simulink model "DW_MCU_Simulation_Architecture_DualMotor"  (R2018a)
settings: Solver=FixedStepDiscrete  StartTime=0.0  StopTime=20  FixedStep=TimeSteps.ModelStep  RelTol=1e-6
PreLoadFcn:
  | addpath('tools');
  | addpath('tools\Config_UI');
  | addpath('tools\support');
  | addpath('tools\FMIKit_for_Simulink');
  | addpath('tools\FMIKit_for_Simulink\slx');
  | addpath('tools\SpeedCommand');
  | addpath('tools\SpeedCommand\exe');
  | addpath('tools\SpeedCommand\view');
  | addpath('tools\MciAPI');
  | addpath('tools\MciAPI\exe');
  | addpath('tools\MciAPI\exe\enums');
  | addpath('tools\Read_PDB_File');
  | addpath('tools\Read_PDB_File\exe');
  | addpath('tools\PILComm');
  | addpath('tools\PILComm\exe');
  | 
  | addpath('exe');
  | addpath('source\c_code');
  | addpath('source\simulink\PlantModels\Sensor');
  | addpath('source\simulink\PlantModels\Rectifiers');
  | addpath('source\simulink\PlantModels\Motors\CIM');
  | addpath('source\simulink\PlantModels\Motors\BPM');
  | addpath('source\simulink\PlantModels\Motors\BPM\SFunctions\10k\Dyno');
  | addpath('source\simulink\PlantModels\Motors\BPM\SFunctions\10k\HA');
  | addpath('source\simulink\PlantModels\Motors\BPM\SFunctions\10k\VA_Agitation');
  | addpath('source\simulink\PlantModels\Motors\BPM\SFunctions\10k\VA_Spin');
  | addpath('source\simulink\PlantModels\Motors\BPM\SFunctions\16k\Dyno');
  | addpath('source\simulink\PlantModels\Motors\BPM\SFunctions\16k\HA');
  | addpath('source\simulink\PlantModels\Motors\BPM\SFunctions\16k\VA_Agitation');
  | addpath('source\simulink\PlantModels\Motors\BPM\SFunctions\16k\VA_Spin');
  | addpath('source\simulink\PlantModels\Inverter');
  | 
  | 
  | addpath('exported_models');
  | clear all;
  | 
  | try
  | FMIKit.initialize()
  | catch
  | display('FMI Kit Initialization Skipped');
  | end
  | 
  | Sim_Arch_Config_UI_App;
PostLoadFcn:
  | myws = get_param(gcs, 'modelworkspace');
  | myws.clear;
  | clear myws;
  | evalin('base', 'recompile_mcu_sim_arch = 1;');
  | updateModelWS(gcs);
InitFcn:
  | if (evalin('base', 'exist(''smlarch_need_reset'') == 1'))
  |     msgbox('Reload Variables before Running');
  |     set_param(gcs, 'SimulationCommand', 'stop');
  | end
  | BusInit;
  | if(  (exist('SimArchUID')) && (strcmp(SimArchUID, 'a') == 1)  )
  |     updateModelWS(gcs);
  | end
  | useModelWS(gcs);
  | Simulink.sdi.close;
model workspace (MAT data in the model file):
  DC_Bus.Const_Vbus = 325
  InputCircuit.R_line = 0.62
  InputCircuit.L_line = 5e-05
  InputCircuit.C_buscap = 8.2e-05
  InputCircuit.R_diode = 0.22
  InputCircuit.R_buscap = 3.235
  InputCircuit.V_knee = 0.64
  InputCircuit.G_off = 3e-09
  InputCircuit.L_pfc = 0
  InputCircuit.R_pfc = 0
  InputCircuit.Vr = 230
  InputCircuit.Vdc_i = 325
  InputCircuit.freq = 50
  InputCircuit.C1 = -0.6111111111
  InputCircuit.C2 = 1.715258789
  InputCircuit.Cvolt = 0.007695895522
  InputCircuit.Vcc = 3.3
  InputCircuit.ADCBit = 12
  Mechanical.belt_ratio = 10
  Mechanical.JDrum = 0.001
  Mechanical.damp = 0
  Mechanical.m_unb = 0
  Mechanical.r_unb = 0
  Mechanical.M_D = 1
  Mechanical.M = 0.2
  Mechanical.R_Drum = 0.254
  Mechanical.R_J = 0.05
  Mechanical.CF = 0
  Motor.Electrical.Rs_a_Ref = 40.5
  Motor.Electrical.Rs_b_Ref = 40.5
  Motor.Electrical.Rs_c_Ref = 40.5
  Motor.Electrical.p_Pole_Pairs = 1
  Motor.Electrical.PM_Flux_f01 = 0.089
  Motor.Electrical.PM_Flux_f02 = 0
  Motor.Electrical.PM_Flux_f03 = 0
  Motor.Electrical.PM_Flux_f04 = 0
  Motor.Electrical.PM_Flux_f05 = 0
  Motor.Electrical.PM_Flux_f06 = 0
  Motor.Electrical.PM_Flux_f07 = 0
  Motor.Electrical.PM_Flux_f08 = 0
  Motor.Electrical.PM_Flux_f09 = 0
  Motor.Electrical.PM_Flux_f10 = 0
  Motor.Electrical.PM_Flux_f11 = 0
  Motor.Electrical.PM_Flux_f12 = 0
  Motor.Electrical.PM_Flux_f13 = 0
  Motor.Electrical.ajust = 1.57
  Motor.Electrical.alpha_s = 0
  Motor.Mechanical.Jrotor = 2e-05
  Motor.Mechanical.B = 0.0002
  Motor.Mechanical.Jadd = 0
  Motor.Mechanical.Rs_Temperature_Ref = 22
  Motor.Mechanical.PM_Temperature_Ref = 22
  Motor.Mechanical.TR = 1
  Motor.Power_Loss.Rot_Loss_Flag = 0
  Motor.Power_Loss.Rot_Loss_Speed0 = 0
  Motor.Power_Loss.Rot_Loss_Speed1 = 500
  Motor.Power_Loss.Rot_Loss_Speed2 = 3000
  Motor.Power_Loss.Rot_Loss_Speed3 = 4000
  Motor.Power_Loss.Rot_Loss_Speed4 = 4000
  Motor.Power_Loss.Rot_Loss_Speed5 = 4000
  Motor.Power_Loss.Rot_Loss_Speed6 = 4000
  Motor.Power_Loss.Rot_Loss_Speed7 = 4000
  Motor.Power_Loss.Rot_Loss_Power0 = 0
  Motor.Power_Loss.Rot_Loss_Power1 = 0
  Motor.Power_Loss.Rot_Loss_Power2 = 0
  Motor.Power_Loss.Rot_Loss_Power3 = 0
  Motor.Power_Loss.Rot_Loss_Power4 = 0
  Motor.Power_Loss.Rot_Loss_Power5 = 0
  Motor.Power_Loss.Rot_Loss_Power6 = 0
  Motor.Power_Loss.Rot_Loss_Power7 = 0
  Motor.Inductance_Variation.Ld_a0 = 0.14
  Motor.Inductance_Variation.Ld_a1 = 0.14
  Motor.Inductance_Variation.Ld_a2 = 0.14
  Motor.Inductance_Variation.Ld_a3 = 0.14
  Motor.Inductance_Variation.Ld_a4 = 0.14
  Motor.Inductance_Variation.Ld_a5 = 0.14
  Motor.Inductance_Variation.Ld_a6 = 0.14
  Motor.Inductance_Variation.Ld_a7 = 0.14
  Motor.Inductance_Variation.Lq_b0 = 0.14
  Motor.Inductance_Variation.Lq_b1 = 0.14
  Motor.Inductance_Variation.Lq_b2 = 0.14
  Motor.Inductance_Variation.Lq_b3 = 0.14
  Motor.Inductance_Variation.Lq_b4 = 0.14
  Motor.Inductance_Variation.Lq_b5 = 0.14
  Motor.Inductance_Variation.Lq_b6 = 0.14
  Motor.Inductance_Variation.Lq_b7 = 0.14
  Motor.Inductance_Variation.I_pk0 = 0
  Motor.Inductance_Variation.I_pk1 = 1
  Motor.Inductance_Variation.I_pk2 = 2
  Motor.Inductance_Variation.I_pk3 = 3
  Motor.Inductance_Variation.I_pk4 = 4
  Motor.Inductance_Variation.I_pk5 = 5
  Motor.Inductance_Variation.I_pk6 = 6
  Motor.Inductance_Variation.I_pk7 = 7
  Paths.complete_file_R = 'settings\ParametersFiles\Rectifier_Parameters\HVPS_230VPFC\DEA703ASIA_AC230V.xml'
  Paths.complete_file_M = 'settings\ParametersFiles\Motor_Parameters\BPM\sBPM\BPM_Aweco_Vsm_Dw03g_Wash_Pump.xml'
  Paths.complete_file_mc = 'settings\ParametersFiles\Mechanical_Parameters\HA\Mechanical_HA.xml'
  Paths.chosen_dir_M = 'settings\ParametersFiles\Motor_Parameters\BPM\sBPM'
  Paths.Setting_File_Path = 'C:\Data\Nucleus_Motor_Control\Dea703_Mcu_Nucleus_Blac_Dev\exe\T40464433_EMEA.bin'
  Paths.Root_Path = 'C:\Data\Nucleus_Motor_Control\Dea703_Mcu_Nucleus_Blac_Dev\source'
  Paths.Object_Path = ''
  Thermal.Tstator = 22
  Thermal.Trotor = 22
  TimeSteps.ModelStep = 0.0001
  TimeSteps.InputCircuitStep = 0.0005
  Variant_Input_Circuit = 5
  Variant_Motor = 3
  Variant_Motor_Control = 1
  Variant_Sensor = 0
  config.MCI_Sampling_Frequency = 'Set'
  config.rect_flag = 0
  config.const_dcbus_flag = 1
  config.Root_Path_flag = 'Source Selected'
  config.Motor_Control_Source = 'Set'
  config.Control_Layer = 'SIL'
  config.Fast_ADC_Initialization_Flag = 'Set'
  config.Skip_Motor_Moving_Handler_Flag = 'Set'
  config.BoardVariant = 'AC230VPFC'
  config.MotorVariant = 'BPM_Leili_Vsm_Dw03g_Drain_Pump'
  config.MechanicalVariant = 'DynoLoad'
  config.Setting_File_Flag = 'Set'
undefined symbols (not defined in the file): DualMotor, Load_D, Load_W, sigbuilder_block, steps
libraries: pdb_libbrowser x7, bpm_dq_S_noH_D_RL_Dyno x2, mciapi_libbrowser x1
(part 1 of 2)
CloseFcn:
  | rmpath('support');
  | rmpath('Compile Scripts');
  | rmpath(genpath('Plant Models'));
  | rmpath(genpath('MciAPI'));
  | clc;
  | clear all;
settings Model: Creator=consul.marchionne  LastModifiedBy=BEATOA
settings DataIOCC: LimitDataPoints=on
settings OptimizationCC: LifeSpan=inf
settings DebuggingCC: SolverPrmCheckMsg=warning  SFUnexpectedBacktrackingDiag=warning  SFNoUnconditionalDefaultTransitionDiag=warning  SFExecutionAtInitializationDiag=none
settings HardwareCC: ProdBitPerPointer=32  ProdBitPerSizeT=32  ProdBitPerPtrDiffT=32  ProdLargestAtomicFloat=None  ProdIntDivRoundTo=Undefined  ProdEndianess=Unspecified  ProdWordSize=32  ProdHWDeviceType=32-bit Generic
settings ModelReferenceCC: UpdateModelReferenceTargets=IfOutOfDate  EnableRefExpFcnMdlSchedulingChecks=off  ModelReferenceNumInstancesAllowed=Single  ModelReferenceMinAlgLoopOccurrences=on  PropagateSignalLabelsOutOfModel=off
settings CodeAppCC: StateflowObjectComments=on
settings GRTTargetCC: TargetLangStandard=C89/C90 (ANSI)  GeneratePreprocessorConditionals=Disable all
settings ConfigComp: CovMetricSettings=dw  CovHtmlReporting=on  CovSaveCumulativeToWorkspaceVar=on  CovSaveSingleToWorkspaceVar=on  CovExternalEMLEnable=off  CovSFcnEnable=off

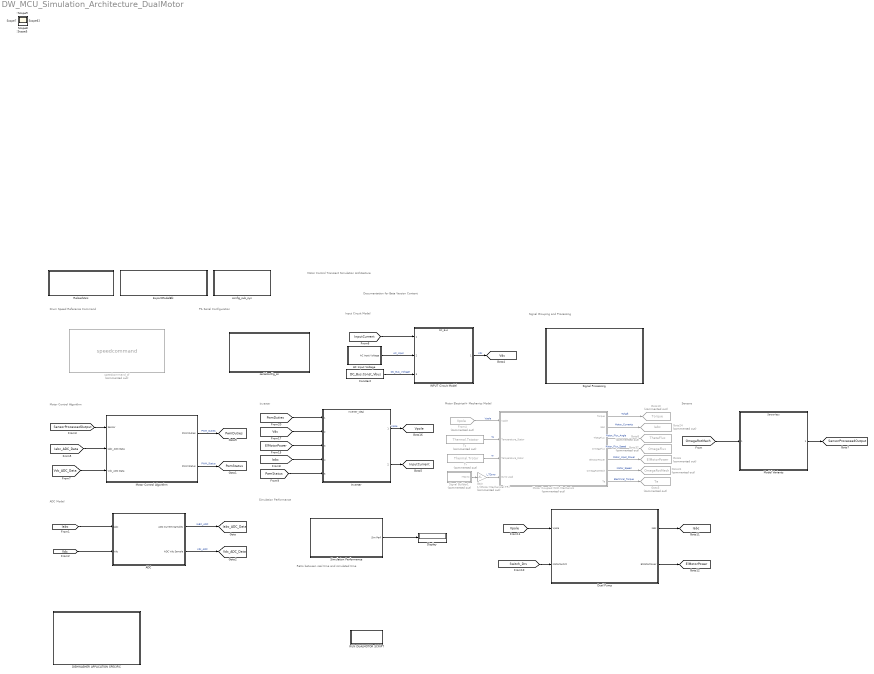
== system DW_MCU_Simulation_Architecture_DualMotor ==
  note: Motor Control Transient Simulation Architecture
  note: Input Circuit Model
  note: Simulation Performance
  note: Ratio between real time and simulated time
  note: ADC Model
  note: Motor Electrical+ Mechanics Model
  note: Inverter
  note: Signal Grouping and Processing
  note: PIL Serial Configuration
  note: Motor Control Algorithm
  note: Sensors
  note: Drum Speed Reference Command
  note: Documentation for Beta Version Content
  AC Input Voltage : Subsystem
  ADC : Subsystem  mask{C1=InputCircuit.C1, C2=InputCircuit.C2, Cvolt=InputCircuit.Cvolt, ADCBit=InputCircuit.ADCBit, Vcc=InputCircuit.Vcc}
  Constant : Constant  Value=DC_Bus.Const_Vbus
  DISHWASHER APPLICATION SPECIFIC : Subsystem
  Display : Display
  Dual Pump : Subsystem  SystemSampleTime=0.000125
      settings: CopyFcn=|
      | blockname = gcb;
      |  linkstatus = lower(get_param(blockname,'LinkStatus'));
      | if strcmp(linkstatus,'resolved')
      |   set_param(gcb,'LinkStatus','none');
      | end
  ExportModelBlk : Subsystem  LoadFcn=|  mask{model_name=}
      | msk = Simulink.Mask.get(gcb);
      | bHandle = msk.getDialogControl('Control2');
      | bHandle.Enabled = 'on';
      | clear msk;
      | clear bHandle;
      mask prompts: model_name "Model's export name (no extension)"
      mask DialogControl Control2 Prompt: Export
      mask DialogControl Control2 Callback:
      | save_system('MCU_Simulation_Architecture');
      | if (strcmp(get_param(gcb, 'model_name'),'') == 1)
      |     msgbox('Must give a name to the model');
      | else
      |     exportSimArch(get_param(gcb, 'model_name'));
      | end
      mask Display: disp('Export current configuration');
  From4 : From  Commented=on  GotoTag=Vpole  TagVisibility=global
  Gain : Gain  Commented=on  Gain=1/(Motor.Mechanical.TR)
  Goto10 : Goto  Commented=on  GotoTag=Torque  TagVisibility=global
  Goto24 : Goto  Commented=on  GotoTag=Iabc  TagVisibility=global
  Goto3 : Goto  Commented=on  GotoTag=Te  TagVisibility=global
  Goto31 : Goto  Commented=on  GotoTag=OmegaRotMech  TagVisibility=global
  Goto32 : Goto  Commented=on  GotoTag=OmegaFlux  TagVisibility=global
  Goto6 : Goto  Commented=on  GotoTag=ElMotorPower  TagVisibility=global
  Goto8 : Goto  Commented=on  GotoTag=ThetaFlux  TagVisibility=global
  INPUT Circuit Model : ModelReference  ModelNameDialog=DC_Bus.slx  SimulationMode=Normal  Variant=on  ModelReferenceVersion=1.7
      settings: AttributesFormatString=%<ActiveVariant>
  Inverter : ModelReference  ModelNameDialog=Inverter_Ideal.slx  SimulationMode=Normal  Variant=on  OverrideUsingVariant=Variant1  ModelReferenceVersion=1.14
      settings: AttributesFormatString=%<ActiveVariant>
  Model Variants : ModelReference  ModelNameDialog=Sensorless.slx  SimulationMode=Normal  Variant=on  ModelReferenceVersion=1.8
      settings: AttributesFormatString=%<ActiveVariant>
  Motor Control Algorithm : Subsystem  SystemSampleTime=6.25e-5
  Motor Coupled With Mechanics : Subsystem  Commented=on  SystemSampleTime=0.000125
      settings: CopyFcn=|
      | blockname = gcb;
      |  linkstatus = lower(get_param(blockname,'LinkStatus'));
      | if strcmp(linkstatus,'resolved')
      |   set_param(gcb,'LinkStatus','none');
      | end
  RUN DUALMOTOR SCRIPT : Subsystem
      settings: AttributesFormatString=|
      | to be executed once, after selecting
      | the sfun motor plant with dyno and
      | before running the simulation for the
      | first time.
      settings: OpenFcn=|
      | addpath('source/simulink')
      | addpath('source')
      | DualMotorScript
  ReloadVars : Subsystem
      settings: OpenFcn=|
      | evalin('base', 'clear smlarch_need_reset');
      | useModelWS(gcs);
      mask Display: disp('Reload Variables');
  Signal Builder1 : Subsystem  Tag=STV Subsys  Commented=on  LoadFcn=sigbuilder_block('load');  StartFcn=sigbuilder_block('start');  StopFcn=sigbuilder_block('stop');  ClipboardFcn=sigbuilder_block('clipboard');  mask(Sigbuilder block){tuvar=[0:10]}
      mask help: Simulink:masks:SigbuilderBlock_MD
      mask init:
      | if ~strcmp(get_param(bdroot(gcbh),'SimulationStatus'),'stopped') tuvar = sigbuilder_block('maskInit'); end
      settings: CopyFcn=sigbuilder_block('copy');  DeleteFcn=sigbuilder_block('delete');  ModelCloseFcn=sigbuilder_block('modelClose');  PreSaveFcn=sigbuilder_block('preSave');  PauseFcn=sigbuilder_block('pause');  ContinueFcn=sigbuilder_block('continue');  NameChangeFcn=sigbuilder_block('namechange');  OpenFcn=sigbuilder_block('open',[199.5 49.5 461.25 300 ]);  CloseFcn=sigbuilder_block('close');
      mask Display: plot(0, 0, 100, 100,[2, 2, 32, 32, 2], [68, 8, 8, 68, 68],[32, 2], [38, 38], [32, 19, 2],[53, 60, 44], [32, 17, 17, 2],[16, 16, 31, 31]);txt = getActiveGroup(gcbh);text(2, 100, txt,'verticalAlignment', 'top');
  Signal Processing : Subsystem
  Simulation Performance : Subsystem
  Tr : Constant  Commented=on  Value=Thermal.Trotor
  Ts : Constant  Commented=on  Value=Thermal.Tstator
  config_sub_sys : Subsystem  TreatAsAtomicUnit=on  mask{mcu_recompile=on}
      mask prompts: mcu_recompile "Recompile"
      mask Display:
      | if (strcmp(get_param(gcb, 'mcu_recompile'),'off') == 1)
      |     disp('Do not Recompile');
      | else
      |     disp('Recompile');
      | end
  serialconfig_ss : Subsystem  mask{comdevtype=RS232, com_port=COM4, baudrate=57600}
      mask prompts: comdevtype "COM Type"; com_port "COM Port"
      mask TypeOptions comdevtype: RS232 | SPI
      mask Callback comdevtype:
      | maskStr = get_param(gcb,'comdevtype');
      | if strcmp(maskStr,'SPI')
      |     assignin('base', 'VARIANT_PIL_COMM', 2);
      | else
      |     assignin('base', 'VARIANT_PIL_COMM', 1);
      | end
      | clear maskStr;
      mask TypeOptions com_port: COM3 | COM4
      mask TypeOptions baudrate: 2400 | 4800 | 9600 | 19200 | 28800 | 38400 | 57600 | 115200 | 230400
      mask DialogControl ParameterGroupVar Prompt: RS232 Settings
      mask DialogControl rfrsh_button Prompt: Refresh Ports
      mask DialogControl rfrsh_button Callback:
      | devices = winqueryreg('name', 'HKEY_LOCAL_MACHINE', 'HARDWARE\DEVICEMAP\SERIALCOMM');
      | if (isempty(devices))
      |     com{1} = 'NONE';
      | else
      |     com = cell(1, length(devices));
      |    % h = waitbar(0,'Scanning Serial Ports...','Name','Scanning Serial Ports...');
      |     for i = 1:length(devices)
      |         com{i} = winqueryreg('HKEY_LOCAL_MACHINE', 'HARDWARE\DEVICEMAP\SERIALCOMM', devices{i});
      |     %    waitbar(i/length(devices),h);
      |     end
      | end
      | 
      | msk = Simulink.Mask.get(gcb);
      | p = msk.Parameters;
      | p(2).TypeOptions = com;
      | clear msk;
      | clear p;
      | clear com;
      | clear devices;
      mask Display: disp('Serial Configuration');
  speedcommand_sf : S-Function  Commented=on  InitFcn=|  StopFcn=|  FunctionName=speedcommand  Parameters=steps, Variant_Motor_Control  SFunctionDeploymentMode=off  EnableBusSupport=off
      InitFcn=|
      | transmission = evalin('base','Motor.Mechanical.TR');
      | if isempty(get_param(gcb,'UserData'))
      | steps = [];
      | else
      |     ud = get_param(gcb,'UserData');
      |     [pts,steps] = GenPlotCmds(ud.table);
      |     for i = 1:size(steps,1)
      |         steps(i,1) = steps(i,1) * transmission;
      |         steps(i,2) = steps(i,2) * transmission;
      |     end
      | end
      | clear transmission;
      | clear i;
      | clear ud;
      StopFcn=|
      | clear steps;
      | clear pts;
      settings: OpenFcn=SpeedCommandView;
  Scope{,2..12} (12 alike) : Scope
  tag scope: ElMotorPower=global, Iabc=global, Iabc_ADC_Data=global, InputCurrent=global, PwmDuties=global, PwmStatus=global, SensorProcessedOutput=global, Vdc=global, Vdc_ADC_Data=global, Vpole=global
  wires:
  [OmegaRotMech] -> Model Variants/1
  Simulation Performance/1(Sim Perf) -> Display/1
  From4/1 -> Motor Coupled With Mechanics/1(Vpole)  "Vpole"
  Motor Coupled With Mechanics/1(Torque) -> Goto10/1  "Tshaft"
  Motor Coupled With Mechanics/2(Iabc) -> Goto24/1  "Motor_Currents"
  Motor Coupled With Mechanics/3(ThetaFlux) -> Goto8/1  "Rotor_Flux_Angle"
  Motor Coupled With Mechanics/4(OmegaFlux) -> Goto32/1  "Rotor_Flux_Speed"
  Motor Coupled With Mechanics/5(ElMotorPower) -> Goto6/1  "Motor_Input_Power"
  Motor Coupled With Mechanics/6(OmegaRotMech) -> Goto31/1  "Motor_Speed"
  [PwmDuties] -> Inverter/1
  [Vdc] -> Inverter/2
  [ElMotorPower] -> Inverter/3
  [Iabc] -> Inverter/4
  Inverter/1 -> [Vpole]  "Vpole"
  Inverter/2 -> [InputCurrent]
  Motor Control Algorithm/1(PWM Duties) -> [PwmDuties]  "PWM_Duties"
  Motor Control Algorithm/2(PWM Status) -> [PwmStatus]  "PWM_Status"
  [SensorProcessedOutput] -> Motor Control Algorithm/1(Sensor)
  INPUT Circuit Model/1 -> [Vdc]  "Vdc"
  Constant/1 -> INPUT Circuit Model/3  "DC_Bus_Voltage"
  AC Input Voltage/1(AC Input Voltage) -> INPUT Circuit Model/2  "AC_Input"
  [InputCurrent] -> INPUT Circuit Model/1
  Model Variants/1 -> [SensorProcessedOutput]
  [PwmStatus] -> Inverter/5
  [Vdc] -> ADC/2(Vdc)
  [Iabc] -> ADC/1(Iabc)
  [Iabc_ADC_Data] -> Motor Control Algorithm/2(Iabc_ADC Data)
  ADC/1(ADC Current Samples) -> [Iabc_ADC_Data]  "IABC_ADC"
  ADC/2(ADC Vdc Sample) -> [Vdc_ADC_Data]  "Vdc_ADC"
  [Vdc_ADC_Data] -> Motor Control Algorithm/3(Vdc_ADC Data)
  Ts/1 -> Motor Coupled With Mechanics/2(Temperature_Stator)  "Ts"
  Tr/1 -> Motor Coupled With Mechanics/3(Temperature_Rotor)  "Tr"
  Gain/1 -> Motor Coupled With Mechanics/4(Dyno Load)  "i_TDyno"
  Signal Builder1/1(iTDyno) -> Gain/1
  Motor Coupled With Mechanics/7(Te) -> Goto3/1  "Electrical_Torque"
  [Switch_Drv] -> Dual Pump/2(MotorSwitch)
  [Vpole] -> Dual Pump/1(Vpole)
  Dual Pump/1(Iabc) -> [Iabc]
  Dual Pump/2(ElMotorPower) -> [ElMotorPower]

== system DW_MCU_Simulation_Architecture_DualMotor/AC Input Voltage ==
  Sine Wave : Sin  Amplitude=InputCircuit.Vr*sqrt(2)  Frequency=InputCircuit.freq*2*pi
  AC Input Voltage : Outport
  wires:
  Sine Wave/1 -> AC Input Voltage/1

== system DW_MCU_Simulation_Architecture_DualMotor/ADC ==
  Iabc : Inport
  Vdc : Inport  Port=2
  ADC Raw : MATLAB Function  TreatAsAtomicUnit=on  mask{C1=C1, C2=C2, Cvolt=Cvolt, ADCBit=ADCBit, Vcc=Vcc}
      mask init:
      | C1=C1;
      | C2=C2;
      | Cvolt=Cvolt;
      | ADCBit=ADCBit;
      | Vcc=Vcc;
  ADC Current Samples : Outport
  ADC Vdc Sample : Outport  Port=2
  wires:
  Iabc/1 -> ADC Raw/1(Iabc)
  Vdc/1 -> ADC Raw/2(Vdc)
  ADC Raw/1(Iabc_samples) -> ADC Current Samples/1
  ADC Raw/2(Vdc_sample) -> ADC Vdc Sample/1

== system DW_MCU_Simulation_Architecture_DualMotor/DISHWASHER APPLICATION SPECIFIC ==
  Clock : Clock
  Constant : Constant  Value=2500
  Demux : Demux
  MATLAB Function : MATLAB Function  TreatAsAtomicUnit=on
  Subsystem : Subsystem
  Unit Delay : UnitDelay  SampleTime=-1
  motorswitch : MATLAB Function  TreatAsAtomicUnit=on
  tag scope: IPM_Temp_ADC=global, Switch_Fbk=global
  wires:
  Constant/1 -> [IPM_Temp_ADC]
  [Switch_Drv] -> motorswitch/1(u)
  motorswitch/1(y) -> Unit Delay/1
  Unit Delay/1 -> [Switch_Fbk]
  Demux/3 -> Subsystem/2(Speed (RPM))
  Demux/4 -> Subsystem/3(Acceleration (RPM/s))
  Demux/1 -> Subsystem/Trigger
  Demux/2 -> Subsystem/1(Load)
  MATLAB Function/1(y) -> Demux/1
  Clock/1 -> MATLAB Function/1(t)

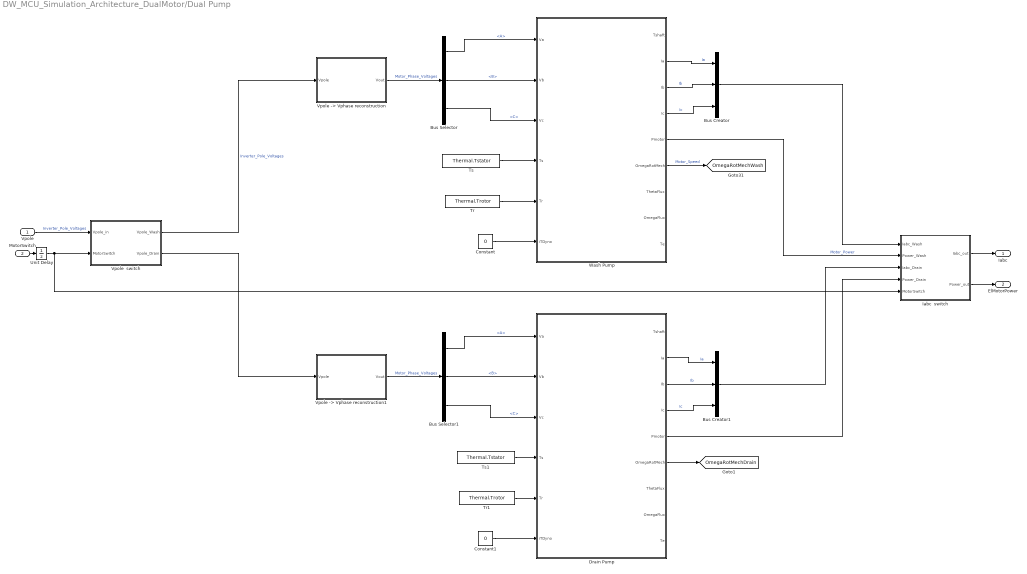
== system DW_MCU_Simulation_Architecture_DualMotor/Dual Pump ==
  Vpole : Inport  OutDataTypeStr=Bus: XabcBus
  MotorSwitch : Inport  Port=2
  Bus Creator : BusCreator  Inputs=3
  Bus Creator1 : BusCreator  Inputs=3
  Bus Selector : BusSelector  OutputSignals=A,B,C
  Bus Selector1 : BusSelector  OutputSignals=A,B,C
  Constant : Constant  Value=0
  Constant1 : Constant  Value=0
  Drain Pump : Subsystem  VariantControl=Variant_Motor_Model_Executable == 3
  Iabc  switch : MATLAB Function  TreatAsAtomicUnit=on
  Tr : Constant  Value=Thermal.Trotor
  Tr1 : Constant  Value=Thermal.Trotor
  Ts : Constant  Value=Thermal.Tstator
  Ts1 : Constant  Value=Thermal.Tstator
  Unit Delay : UnitDelay  SampleTime=-1
  Vpole  switch : MATLAB Function  TreatAsAtomicUnit=on
  "Vpole -> Vphase reconstruction" : MATLAB Function  TreatAsAtomicUnit=on
  "Vpole -> Vphase reconstruction1" : MATLAB Function  TreatAsAtomicUnit=on
  Wash Pump : Subsystem  VariantControl=Variant_Motor_Model_Executable == 3
  Iabc : Outport  OutDataTypeStr=Bus: XabcBus
  ElMotorPower : Outport  Port=2
  tag scope: OmegaRotMechDrain=global, OmegaRotMechWash=global
  wires:
  Bus Creator/1 -> Iabc  switch/1(Iabc_Wash)
  Vpole  switch/1(Vpole_Wash) -> "Vpole -> Vphase reconstruction"/1(Vpole)  "Inverter_Pole_Voltages"
  "Vpole -> Vphase reconstruction"/1(Vout) -> Bus Selector/1  "Motor_Phase_Voltages"
  Bus Selector/1 -> Wash Pump/1(Va)  "<A>"
  Bus Selector/2 -> Wash Pump/2(Vb)  "<B>"
  Bus Selector/3 -> Wash Pump/3(Vc)  "<C>"
  Wash Pump/2(Ia) -> Bus Creator/1  "Ia"
  Wash Pump/3(Ib) -> Bus Creator/2  "Ib"
  Wash Pump/4(Ic) -> Bus Creator/3  "Ic"
  Wash Pump/5(Pmotor) -> Iabc  switch/2(Power_Wash)  "Motor_Power"
  Drain Pump/2(Ia) -> Bus Creator1/1  "Ia"
  Bus Creator1/1 -> Iabc  switch/3(Iabc_Drain)
  Drain Pump/4(Ic) -> Bus Creator1/3  "Ic"
  Drain Pump/3(Ib) -> Bus Creator1/2  "Ib"
  Bus Selector1/1 -> Drain Pump/1(Va)  "<A>"
  "Vpole -> Vphase reconstruction1"/1(Vout) -> Bus Selector1/1  "Motor_Phase_Voltages"
  Bus Selector1/2 -> Drain Pump/2(Vb)  "<B>"
  Bus Selector1/3 -> Drain Pump/3(Vc)  "<C>"
  MotorSwitch/1 -> Unit Delay/1
  Vpole/1 -> Vpole  switch/1(Vpole_in)  "Inverter_Pole_Voltages"
  Vpole  switch/2(Vpole_Drain) -> "Vpole -> Vphase reconstruction1"/1(Vpole)
  Iabc  switch/2(Power_out) -> ElMotorPower/1
  Iabc  switch/1(Iabc_out) -> Iabc/1
  Drain Pump/5(Pmotor) -> Iabc  switch/4(Power_Drain)
  Ts/1 -> Wash Pump/4(Ts)
  Ts1/1 -> Drain Pump/4(Ts)
  Tr/1 -> Wash Pump/5(Tr)
  Tr1/1 -> Drain Pump/5(Tr)
  Constant/1 -> Wash Pump/6(iTDyno)
  Constant1/1 -> Drain Pump/6(iTDyno)
  Wash Pump/6(OmegaRotMech) -> [OmegaRotMechWash]  "Motor_Speed"
  Drain Pump/6(OmegaRotMech) -> [OmegaRotMechDrain]
  Unit Delay/1 -> Iabc  switch/5(MotorSwitch), Vpole  switch/2(MotorSwitch)

== system DW_MCU_Simulation_Architecture_DualMotor/ExportModelBlk ==

== system DW_MCU_Simulation_Architecture_DualMotor/Motor Control Algorithm ==
  Sensor : Inport
  Iabc_ADC Data : Inport  Port=2
  Vdc_ADC Data : Inport  Port=3
  Scope : Scope
  WINDY CIM_BPM : Subsystem  Variant=on
  PWM Duties : Outport
  PWM Status : Outport  Port=2
  wires:
  WINDY CIM_BPM/1(Duties) -> PWM Duties/1  "PWM_Duties"
  WINDY CIM_BPM/2(Pwm Status) -> PWM Status/1  "PWM_Status"
  Sensor/1 -> WINDY CIM_BPM/1(Sensor)
  Iabc_ADC Data/1 -> WINDY CIM_BPM/2(Iabc_ADC Data)
  Vdc_ADC Data/1 -> WINDY CIM_BPM/3(Vdc_ADC Data)
  WINDY CIM_BPM/3(CPU Cycles) -> Scope/1

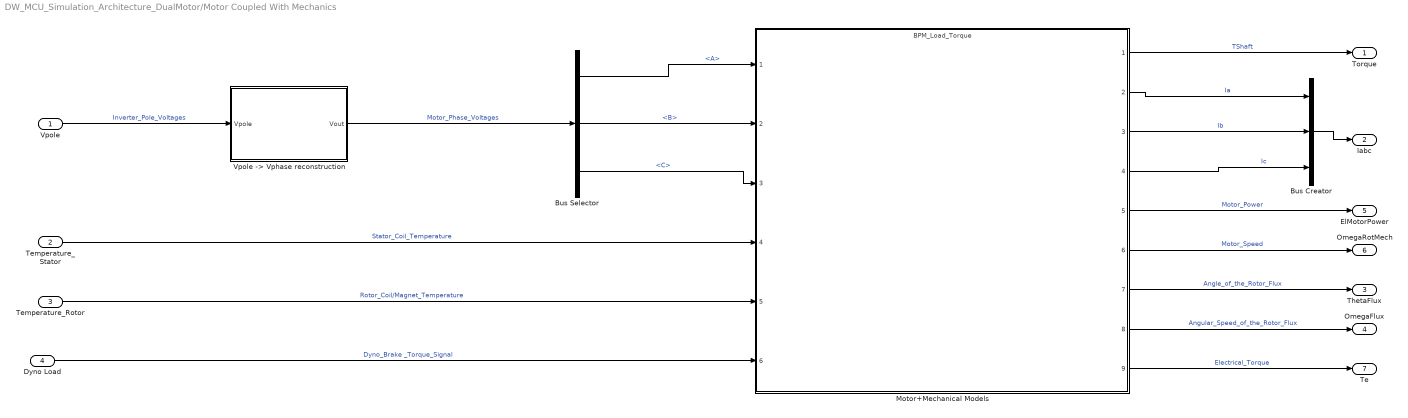
== system DW_MCU_Simulation_Architecture_DualMotor/Motor Coupled With Mechanics ==
  Vpole : Inport  OutDataTypeStr=Bus: XabcBus
  Temperature_Stator : Inport  Port=2
  Temperature_Rotor : Inport  Port=3
  Dyno Load : Inport  Port=4
  Bus Creator : BusCreator  Inputs=3
  Bus Selector : BusSelector  OutputSignals=A,B,C
  Motor+Mechanical Models : ModelReference  ModelNameDialog=BPM_Load_Torque.slx  SimulationMode=Normal  Variant=on  ModelReferenceVersion=1.220
      settings: AttributesFormatString=%<ActiveVariant>
  "Vpole -> Vphase reconstruction" : MATLAB Function  TreatAsAtomicUnit=on
  Torque : Outport
  Iabc : Outport  Port=2  OutDataTypeStr=Bus: XabcBus
  ThetaFlux : Outport  Port=3
  OmegaFlux : Outport  Port=4
  ElMotorPower : Outport  Port=5
  OmegaRotMech : Outport  Port=6
  Te : Outport  Port=7
  wires:
  Bus Creator/1 -> Iabc/1
  Vpole/1 -> "Vpole -> Vphase reconstruction"/1(Vpole)  "Inverter_Pole_Voltages"
  "Vpole -> Vphase reconstruction"/1(Vout) -> Bus Selector/1  "Motor_Phase_Voltages"
  Bus Selector/1 -> Motor+Mechanical Models/1  "<A>"
  Bus Selector/2 -> Motor+Mechanical Models/2  "<B>"
  Bus Selector/3 -> Motor+Mechanical Models/3  "<C>"
  Temperature_Stator/1 -> Motor+Mechanical Models/4  "Stator_Coil_Temperature"
  Temperature_Rotor/1 -> Motor+Mechanical Models/5  "Rotor_Coil/Magnet_Temperature"
  Motor+Mechanical Models/1 -> Torque/1  "TShaft"
  Motor+Mechanical Models/2 -> Bus Creator/1  "Ia"
  Motor+Mechanical Models/3 -> Bus Creator/2  "Ib"
  Motor+Mechanical Models/4 -> Bus Creator/3  "Ic"
  Motor+Mechanical Models/5 -> ElMotorPower/1  "Motor_Power"
  Motor+Mechanical Models/6 -> OmegaRotMech/1  "Motor_Speed"
  Motor+Mechanical Models/7 -> ThetaFlux/1  "Angle_of_the_Rotor_Flux"
  Dyno Load/1 -> Motor+Mechanical Models/6  "Dyno_Brake _Torque_Signal"
  Motor+Mechanical Models/8 -> OmegaFlux/1  "Angular_Speed_of_the_Rotor_Flux"
  Motor+Mechanical Models/9 -> Te/1  "Electrical_Torque"

== system DW_MCU_Simulation_Architecture_DualMotor/RUN DUALMOTOR SCRIPT ==

== system DW_MCU_Simulation_Architecture_DualMotor/ReloadVars ==

== system DW_MCU_Simulation_Architecture_DualMotor/Signal Builder1 ==
  Demux : Demux  Tag=STV Demux  Outputs=1
  FromWs : FromWorkspace  Tag=STV FromWs  VariableName=tuvar  SampleTime=0
      SigBuilderData=|
      | common.afterFinalStr = 'Extrapolate'
      | common.sampleTime = 0
      | dataSet.timeRange = [0 30]
      | dataSet.name = 'Dyno_Load_Profile'
      | sbobj.Groups.Name = 'Dyno_Load_Profile'
      | sbobj.Groups.Signals.Name = 'iTDyno'
      | sbobj.Groups.Signals.XData = [0 0.8 4 20 28 30]
      | sbobj.Groups.Signals.YData = [0 0 0 0 0 0]
      | sbobj.Groups.TimeRange = [0 30]
  iTDyno : Outport  Tag=STV Outport
  wires:
  Demux/1 -> iTDyno/1
  FromWs/1 -> Demux/1

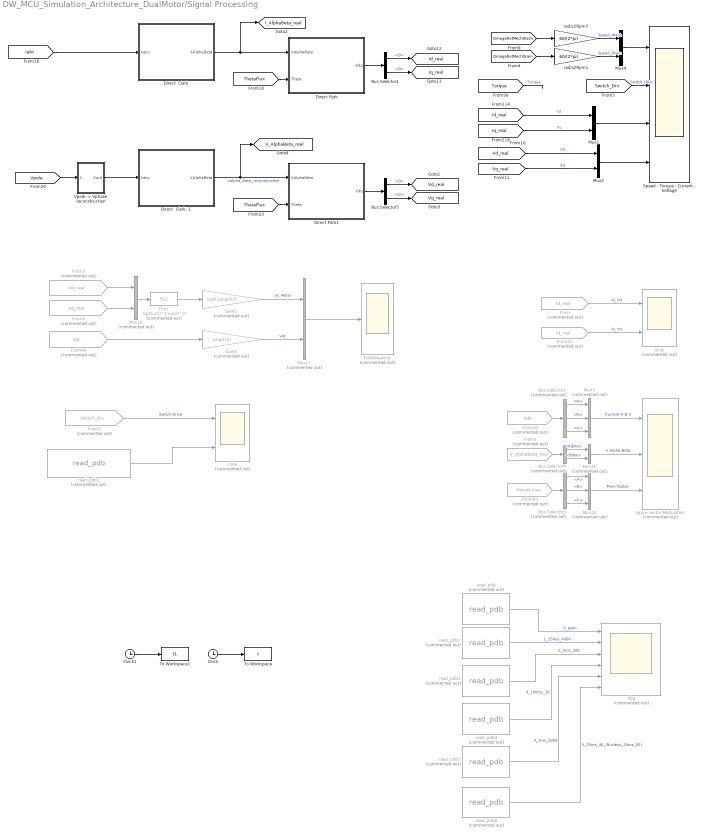
== system DW_MCU_Simulation_Architecture_DualMotor/Signal Processing ==
  Bus Selector1 : BusSelector  OutputSignals=D,Q
  Bus Selector2 : BusSelector  Commented=on  OutputSignals=Ia,Ib,Ic
  Bus Selector3 : BusSelector  Commented=on  OutputSignals=A,B,C
  Bus Selector5 : BusSelector  OutputSignals=D,Q
  Bus Selector6 : BusSelector  Commented=on  OutputSignals=Alpha,Beta
  Clock : Clock
  Clock1 : Clock
  "Direct  Clark  " : MATLAB Function  TreatAsAtomicUnit=on  SystemSampleTime=SystemSampleTime  mask{SystemSampleTime=-1}
      mask prompts: SystemSampleTime "Simulink:blkprm_prompts:AllBlksSampleTime"
  Direct  Clark  1 : MATLAB Function  TreatAsAtomicUnit=on  SystemSampleTime=SystemSampleTime  mask{SystemSampleTime=-1}
      mask prompts: SystemSampleTime "Simulink:blkprm_prompts:AllBlksSampleTime"
  Direct Park : MATLAB Function  TreatAsAtomicUnit=on  SystemSampleTime=SystemSampleTime  mask{SystemSampleTime=-1}
      mask prompts: SystemSampleTime "Simulink:blkprm_prompts:AllBlksSampleTime"
  Direct Park1 : MATLAB Function  TreatAsAtomicUnit=on  SystemSampleTime=SystemSampleTime  mask{SystemSampleTime=-1}
      mask prompts: SystemSampleTime "Simulink:blkprm_prompts:AllBlksSampleTime"
  Fcn1 : Fcn  Commented=on  Expr=sqrt(u(1)^2+u(2)^2)
  "FieldWeaking " : Scope  Commented=on
  From : From  Commented=on  GotoTag=Id_real  TagVisibility=global
  From1 : From  Commented=on  GotoTag=Switch_Drv  TagVisibility=global
  From2 : From  Commented=on  GotoTag=V_AlphaBeta_real  TagVisibility=global
  From3 : From  Commented=on  GotoTag=Vd_real  TagVisibility=global
  From40 : From  Commented=on  GotoTag=Iabc  TagVisibility=global
  From41 : From  Commented=on  GotoTag=Iq_real  TagVisibility=global
  From43 : From  Commented=on  GotoTag=PwmDuties  TagVisibility=global
  From46 : From  Commented=on  GotoTag=Vdc  TagVisibility=global
  From8 : From  Commented=on  GotoTag=Vq_real  TagVisibility=global
  Gain4 : Gain  Commented=on  Gain=1/sqrt(2)
  Gain5 : Gain  Commented=on  Gain=sqrt(3)/sqrt(2)
  Id iq : Scope  Commented=on  NumInputPorts=2
  Mux1 : Mux  Inputs=2
  Mux10 : Mux  Commented=on  Inputs=3
  Mux15 : Mux  Commented=on  Inputs=2
  Mux17 : Mux  Commented=on  Inputs=2
  Mux18 : Mux  Commented=on  Inputs=2
  Mux2 : Mux  Inputs=2
  Mux3 : Mux  Commented=on  Inputs=3
  Mux4 : Mux  Inputs=2
  Speed - Torque - Current - Voltage : Scope  NumInputPorts=4
  To Workspace : ToWorkspace  VariableName=t  SampleTime=-1
      settings: Save2DSignal=2-D array (concatenate along first dimension)
  To Workspace1 : ToWorkspace  VariableName=t1  SampleTime=-1
      settings: Save2DSignal=2-D array (concatenate along first dimension)
  "Vpole -> Vphase reconstruction" : MATLAB Function  TreatAsAtomicUnit=on
  code : Scope  Commented=on  NumInputPorts=2
  dbg : Scope  Commented=on  NumInputPorts=6
  rad/s2Rpm1 : Gain  Gain=60/(2*pi)
  rad/s2Rpm7 : Gain  Gain=60/(2*pi)
  read_pdb : pdb_libbrowser/read_pdb  Commented=on  vstring=dbg_scheduler_0
      settings: SourceProductName=Sim Arch
  read_pdb1 : pdb_libbrowser/read_pdb  Commented=on  vstring=Command_Manager_State
      settings: SourceProductName=Sim Arch
  read_pdb2 : pdb_libbrowser/read_pdb  Commented=on  vstring=dbg_scheduler_1
      settings: SourceProductName=Sim Arch
  read_pdb3 : pdb_libbrowser/read_pdb  Commented=on  vstring=dbg_scheduler_2
      settings: SourceProductName=Sim Arch
  read_pdb4 : pdb_libbrowser/read_pdb  Commented=on  vstring=dbg_scheduler_3
      settings: SourceProductName=Sim Arch
  read_pdb5 : pdb_libbrowser/read_pdb  Commented=on  vstring=dbg_scheduler_4
      settings: SourceProductName=Sim Arch
  read_pdb6 : pdb_libbrowser/read_pdb  Commented=on  vstring=dbg_scheduler_5
      settings: SourceProductName=Sim Arch
  space vector Modulation : Scope  Commented=on  NumInputPorts=3
  tag scope: I_AlphaBeta_real=global, Id_real=global, Iq_real=global, V_AlphaBeta_real=global, Vd_real=global, Vq_real=global
  wires:
  [OmegaRotMechWash] -> rad/s2Rpm7/1
  [Vq_real] -> Mux2/2  "Vq"
  [Id_real] -> Mux1/1  "Id"
  [Iabc] -> "Direct  Clark  "/1(Xabc)
  Direct Park/1(Xdq) -> Bus Selector1/1
  Bus Selector1/1 -> [Id_real]  "<D>"
  Bus Selector1/2 -> [Iq_real]  "<Q>"
  Fcn1/1 -> Gain5/1
  Mux18/1 -> Fcn1/1
  From3/1 -> Mux18/1
  From8/1 -> Mux18/2
  Mux17/1 -> "FieldWeaking "/1
  From46/1 -> Gain4/1
  Bus Selector3/1 -> Mux10/1  "<A>"
  Bus Selector3/2 -> Mux10/2  "<B>"
  Bus Selector3/3 -> Mux10/3  "<C>"
  Mux10/1 -> space vector Modulation/3  "Pwm Duties"
  Bus Selector2/1 -> Mux3/1  "<Ia>"
  Bus Selector2/2 -> Mux3/2  "<Ib>"
  Bus Selector2/3 -> Mux3/3  "<Ic>"
  From40/1 -> Bus Selector2/1
  From43/1 -> Bus Selector3/1
  "Direct  Clark  "/1(XAlphaBeta) -> [I_AlphaBeta_real], Direct Park/1(XAlphaBeta)
  Clock/1 -> To Workspace/1
  Clock1/1 -> To Workspace1/1
  From/1 -> Id iq/1  "Id_rot"
  From41/1 -> Id iq/2  "Iq_rot"
  Gain4/1 -> Mux17/2  "Vdc"
  Gain5/1 -> Mux17/1  "Vs_Motor"
  Mux3/1 -> space vector Modulation/1  "Current A B C"
  [ThetaFlux] -> Direct Park/2(Theta)
  "Vpole -> Vphase reconstruction"/1(Vout) -> Direct  Clark  1/1(Xabc)
  [Vpole] -> "Vpole -> Vphase reconstruction"/1(Vpole)
  Direct  Clark  1/1(XAlphaBeta) -> Direct Park1/1(XAlphaBeta), [V_AlphaBeta_real]  "Valpha_Beta_reconstructed"
  From2/1 -> Bus Selector6/1
  Bus Selector6/1 -> Mux15/1  "<Alpha>"
  Bus Selector6/2 -> Mux15/2  "<Beta>"
  Mux15/1 -> space vector Modulation/2  "V Alpha Beta"
  Bus Selector5/2 -> [Vq_real]  "<Q>"
  Bus Selector5/1 -> [Vd_real]  "<D>"
  [ThetaFlux] -> Direct Park1/2(Theta)
  Direct Park1/1(Xdq) -> Bus Selector5/1
  [Iq_real] -> Mux1/2  "Iq"
  [Vd_real] -> Mux2/1  "Vd"
  [Torque] -> ?  "Torque"
  Mux2/1 -> Speed - Torque - Current - Voltage/4
  Mux1/1 -> Speed - Torque - Current - Voltage/3
  From1/1 -> code/1  "Switch Drive"
  read_pdb1/1 -> code/2
  read_pdb2/1 -> dbg/2  "1_250us_4000"
  read_pdb3/1 -> dbg/3  "2_5ms_200"
  read_pdb6/1 -> dbg/6  "5_25ms_40_(Nucleus_20ms_50)"
  read_pdb/1 -> dbg/1  "0_pwm"
  read_pdb5/1 -> dbg/5  "4_1ms_1000"
  read_pdb4/1 -> dbg/4  "3_100ms_10"
  rad/s2Rpm7/1 -> Mux4/1  "Speed_Wash"
  [OmegaRotMechDrain] -> rad/s2Rpm1/1
  rad/s2Rpm1/1 -> Mux4/2  "Speed_Drain"
  Mux4/1 -> Speed - Torque - Current - Voltage/1
  [Switch_Drv] -> Speed - Torque - Current - Voltage/2  "Switch_DRV"

== system DW_MCU_Simulation_Architecture_DualMotor/Simulation Performance ==
  Clock : Clock
  MATLAB Function : MATLAB Function  TreatAsAtomicUnit=on
  Sim Perf : Outport
  wires:
  MATLAB Function/1(y) -> Sim Perf/1
  Clock/1 -> MATLAB Function/1(t)

== system DW_MCU_Simulation_Architecture_DualMotor/config_sub_sys ==

== system DW_MCU_Simulation_Architecture_DualMotor/serialconfig_ss ==

== system DW_MCU_Simulation_Architecture_DualMotor/DISHWASHER APPLICATION SPECIFIC/Subsystem ==
  Load : Inport
  Speed (RPM) : Inport  Port=2
  Acceleration (RPM/s) : Inport  Port=3
  Trigger : TriggerPort  VariantControl=Variant  PortDimensions=1
  commandmanager_runload : mciapi_libbrowser/commandmanager_runload  SFunctionModules=''
      settings: SourceProductName=Sim Arch
  Out1 : Outport
  wires:
  commandmanager_runload/1 -> Out1/1
  Load/1 -> commandmanager_runload/1
  Speed (RPM)/1 -> commandmanager_runload/2
  Acceleration (RPM/s)/1 -> commandmanager_runload/3

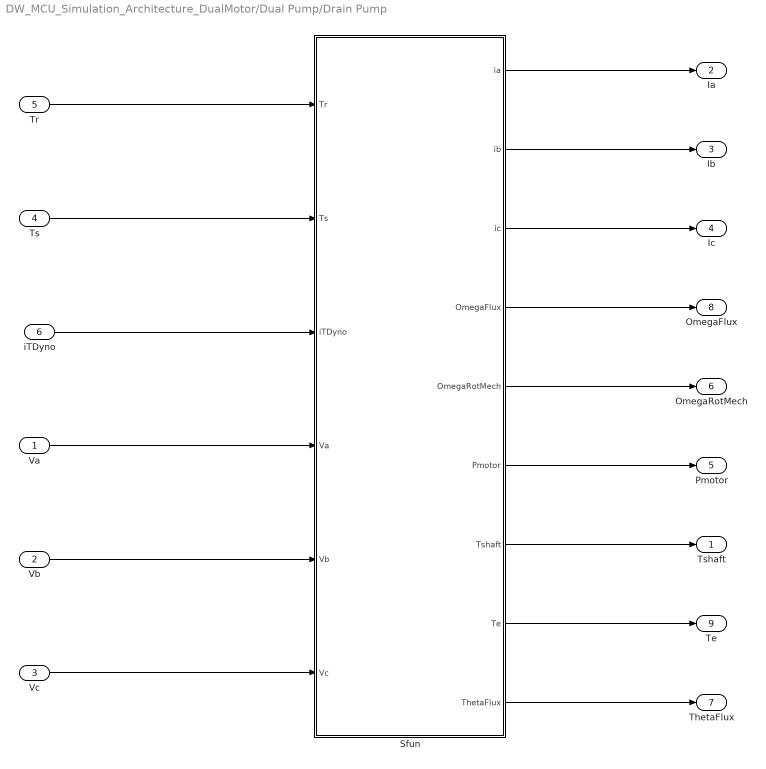
== system DW_MCU_Simulation_Architecture_DualMotor/Dual Pump/Drain Pump ==
  Va : Inport
  Vb : Inport  Port=2
  Vc : Inport  Port=3
  Ts : Inport  Port=4
  Tr : Inport  Port=5
  iTDyno : Inport  Port=6
  Sfun : Subsystem
  Tshaft : Outport
  Ia : Outport  Port=2
  Ib : Outport  Port=3
  Ic : Outport  Port=4
  Pmotor : Outport  Port=5
  OmegaRotMech : Outport  Port=6
  ThetaFlux : Outport  Port=7
  OmegaFlux : Outport  Port=8
  Te : Outport  Port=9
  wires:
  Tr/1 -> Sfun/1(Tr)
  Ts/1 -> Sfun/2(Ts)
  iTDyno/1 -> Sfun/3(iTDyno)
  Va/1 -> Sfun/4(Va)
  Vb/1 -> Sfun/5(Vb)
  Vc/1 -> Sfun/6(Vc)
  Sfun/1(ia) -> Ia/1
  Sfun/2(ib) -> Ib/1
  Sfun/3(ic) -> Ic/1
  Sfun/4(OmegaFlux) -> OmegaFlux/1
  Sfun/5(OmegaRotMech) -> OmegaRotMech/1
  Sfun/6(Pmotor) -> Pmotor/1
  Sfun/7(Tshaft) -> Tshaft/1
  Sfun/8(Te) -> Te/1
  Sfun/9(ThetaFlux) -> ThetaFlux/1

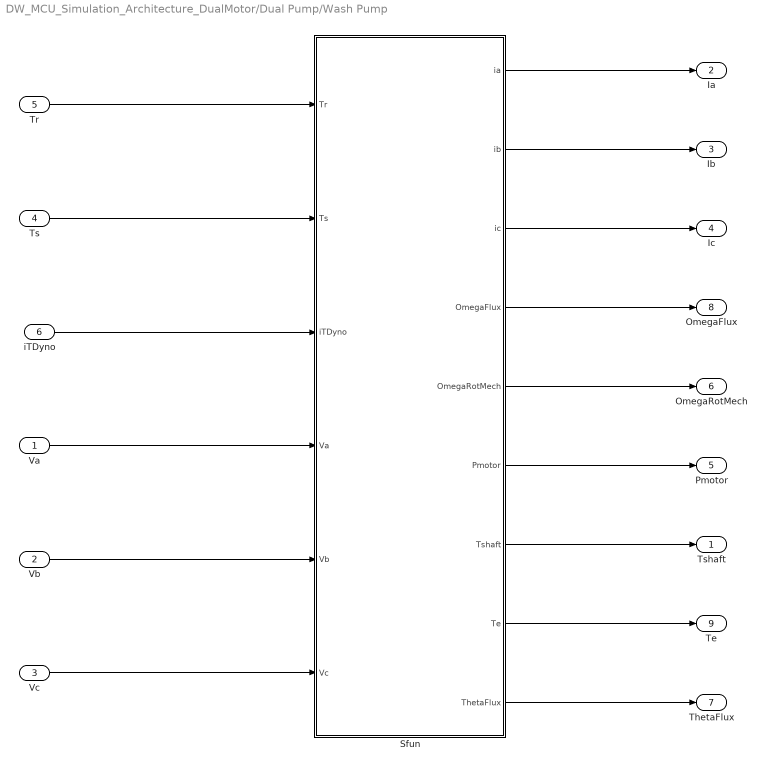
== system DW_MCU_Simulation_Architecture_DualMotor/Dual Pump/Wash Pump ==
  Va : Inport
  Vb : Inport  Port=2
  Vc : Inport  Port=3
  Ts : Inport  Port=4
  Tr : Inport  Port=5
  iTDyno : Inport  Port=6
  Sfun : Subsystem
  Tshaft : Outport
  Ia : Outport  Port=2
  Ib : Outport  Port=3
  Ic : Outport  Port=4
  Pmotor : Outport  Port=5
  OmegaRotMech : Outport  Port=6
  ThetaFlux : Outport  Port=7
  OmegaFlux : Outport  Port=8
  Te : Outport  Port=9
  wires:
  Tr/1 -> Sfun/1(Tr)
  Ts/1 -> Sfun/2(Ts)
  iTDyno/1 -> Sfun/3(iTDyno)
  Va/1 -> Sfun/4(Va)
  Vb/1 -> Sfun/5(Vb)
  Vc/1 -> Sfun/6(Vc)
  Sfun/1(ia) -> Ia/1
  Sfun/2(ib) -> Ib/1
  Sfun/3(ic) -> Ic/1
  Sfun/4(OmegaFlux) -> OmegaFlux/1
  Sfun/5(OmegaRotMech) -> OmegaRotMech/1
  Sfun/6(Pmotor) -> Pmotor/1
  Sfun/7(Tshaft) -> Tshaft/1
  Sfun/8(Te) -> Te/1
  Sfun/9(ThetaFlux) -> ThetaFlux/1

== system DW_MCU_Simulation_Architecture_DualMotor/Motor Control Algorithm/WINDY CIM_BPM ==
  Sensor : Inport
  Iabc_ADC Data : Inport  Port=2
  Vdc_ADC Data : Inport  Port=3
  PIL : Subsystem  InitFcn=|  VariantControl=Variant_Motor_Control==2
      | Control_Layer=evalin('base','config.Control_Layer');
      | 
      | switch Control_Layer
      |    case 'MCI'
      | 
      |      Compile_Link_MCI(config.Root_Path_flag, Paths.Root_Path, config.Motor, Paths.Object_Path)
      | 
      | case 'MCU'
      |    
      |      Compile_Link_MCU(config.Root_Path_flag, Paths.Root_Path, config.Motor, Paths.Object_Path)
      | end
      | 
      | clear Control_Layer;
  SIL : Subsystem  VariantControl=Variant_Motor_Control==1
  Duties : Outport
  Pwm Status : Outport  Port=2
  CPU Cycles : Outport  Port=3

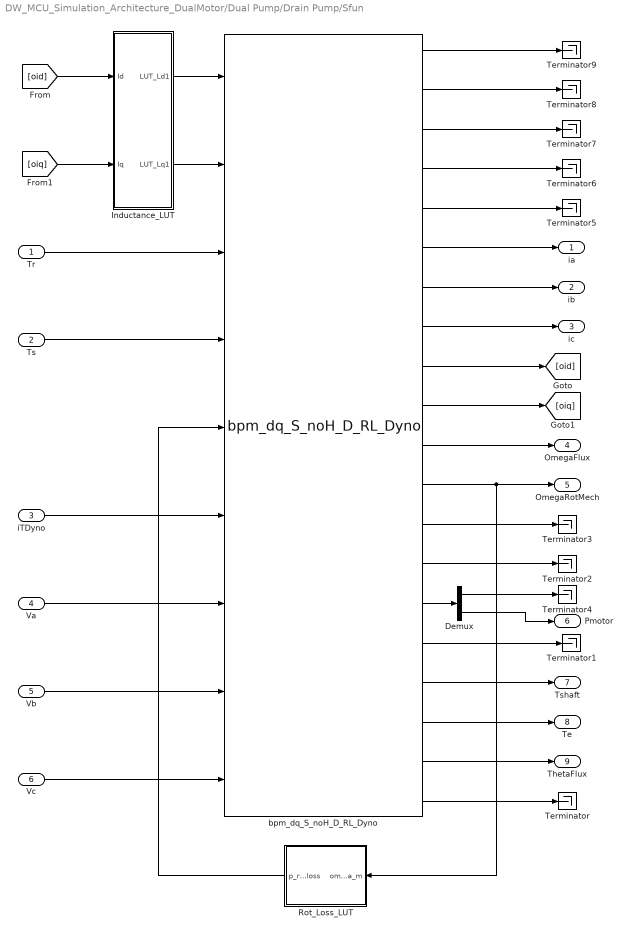
== system DW_MCU_Simulation_Architecture_DualMotor/Dual Pump/Drain Pump/Sfun ==
  Tr : Inport
  Ts : Inport  Port=2
  iTDyno : Inport  Port=3
  Va : Inport  Port=4
  Vb : Inport  Port=5
  Vc : Inport  Port=6
  Demux : Demux  Outputs=2
  Inductance_LUT : Subsystem
  Rot_Loss_LUT : Subsystem
  Terminator{,1..9} (10 alike) : Terminator
  bpm_dq_S_noH_D_RL_Dyno : bpm_dq_S_noH_D_RL_Dyno/bpm_dq_S_noH_D_RL_Dyno  Description=Subsystem: bpm_dq_S_noH_D_RL_Dyno  ic=[0., 0., 0., 0.]  Par1=DualMotor(Load_D).Mechanical.B  Par2=DualMotor(Load_D).Mechanical.Jrotor  Par3=DualMotor(Load_D).Inductance_Variation.Ld_a0  Par4=DualMotor(Load_D).Inductance_Variation.Lq_b0  Par5=2  Par6=DualMotor(Load_D).Electrical.p_Pole_Pairs  Par7=DualMotor(Load_D).Power_Loss.Rot_Loss_Flag  Par8=2  Par9=5  Par10=DualMotor(Load_D).Electrical.Rs_a_Ref  Par11=DualMotor(Load_D).Mechanical.PM_Temperature_Ref  Par12=DualMotor(Load_D).Mechanical.Rs_Temperature_Ref  Par13=DualMotor(Load_D).Electrical.alpha_s  Par14=0.00206  Par15=DualMotor(Load_D).Electrical.PM_Flux_f01  Par16=TimeSteps.ModelStep  Par17=-1.  Par18=-1.  MinStep=1/40
  ia : Outport
  ib : Outport  Port=2
  ic : Outport  Port=3
  OmegaFlux : Outport  Port=4
  OmegaRotMech : Outport  Port=5
  Pmotor : Outport  Port=6
  Tshaft : Outport  Port=7
  Te : Outport  Port=8
  ThetaFlux : Outport  Port=9
  wires:
  bpm_dq_S_noH_D_RL_Dyno/2 -> Terminator8/1
  bpm_dq_S_noH_D_RL_Dyno/1 -> Terminator9/1
  iTDyno/1 -> bpm_dq_S_noH_D_RL_Dyno/6
  Va/1 -> bpm_dq_S_noH_D_RL_Dyno/7
  [oiq] -> Inductance_LUT/2(Iq)
  [oid] -> Inductance_LUT/1(Id)
  bpm_dq_S_noH_D_RL_Dyno/5 -> Terminator5/1
  bpm_dq_S_noH_D_RL_Dyno/7 -> ib/1
  bpm_dq_S_noH_D_RL_Dyno/3 -> Terminator7/1
  bpm_dq_S_noH_D_RL_Dyno/10 -> [oiq]
  bpm_dq_S_noH_D_RL_Dyno/9 -> [oid]
  bpm_dq_S_noH_D_RL_Dyno/8 -> ic/1
  bpm_dq_S_noH_D_RL_Dyno/4 -> Terminator6/1
  Vb/1 -> bpm_dq_S_noH_D_RL_Dyno/8
  Ts/1 -> bpm_dq_S_noH_D_RL_Dyno/4
  Tr/1 -> bpm_dq_S_noH_D_RL_Dyno/3
  bpm_dq_S_noH_D_RL_Dyno/6 -> ia/1
  Vc/1 -> bpm_dq_S_noH_D_RL_Dyno/9
  bpm_dq_S_noH_D_RL_Dyno/11 -> OmegaFlux/1
  bpm_dq_S_noH_D_RL_Dyno/12 -> OmegaRotMech/1, Rot_Loss_LUT/1(omega_m)
  bpm_dq_S_noH_D_RL_Dyno/15 -> Demux/1
  bpm_dq_S_noH_D_RL_Dyno/14 -> Terminator2/1
  bpm_dq_S_noH_D_RL_Dyno/13 -> Terminator3/1
  bpm_dq_S_noH_D_RL_Dyno/16 -> Terminator1/1
  bpm_dq_S_noH_D_RL_Dyno/17 -> Tshaft/1
  bpm_dq_S_noH_D_RL_Dyno/18 -> Te/1
  bpm_dq_S_noH_D_RL_Dyno/20 -> Terminator/1
  bpm_dq_S_noH_D_RL_Dyno/19 -> ThetaFlux/1
  Inductance_LUT/2(LUT_Lq1) -> bpm_dq_S_noH_D_RL_Dyno/2
  Inductance_LUT/1(LUT_Ld1) -> bpm_dq_S_noH_D_RL_Dyno/1
  Rot_Loss_LUT/1(p_rot_loss) -> bpm_dq_S_noH_D_RL_Dyno/5
  Demux/1 -> Terminator4/1
  Demux/2 -> Pmotor/1

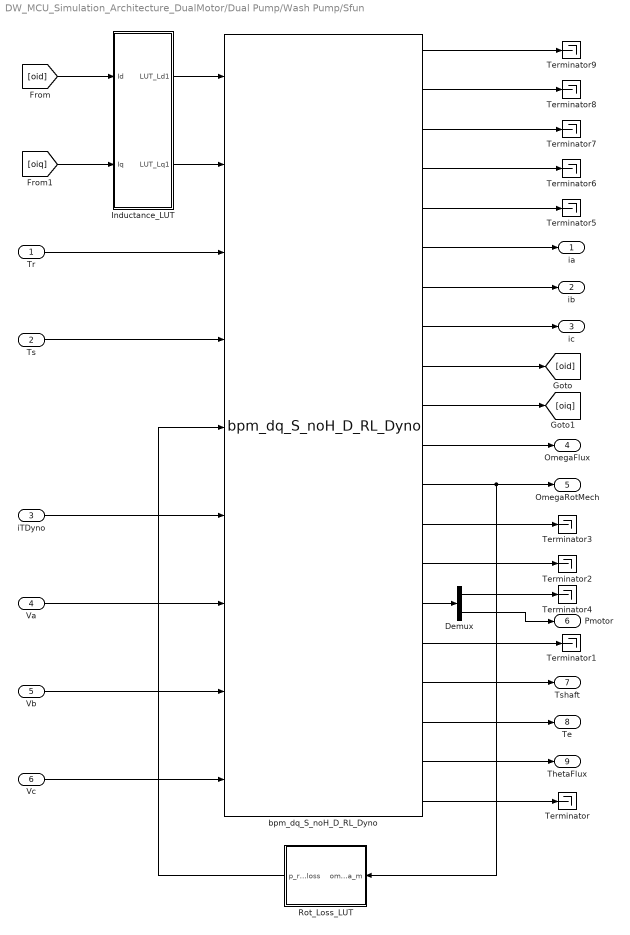
== system DW_MCU_Simulation_Architecture_DualMotor/Dual Pump/Wash Pump/Sfun ==
  Tr : Inport
  Ts : Inport  Port=2
  iTDyno : Inport  Port=3
  Va : Inport  Port=4
  Vb : Inport  Port=5
  Vc : Inport  Port=6
  Demux : Demux  Outputs=2
  Inductance_LUT : Subsystem
  Rot_Loss_LUT : Subsystem
  Terminator{,1..9} (10 alike) : Terminator
  bpm_dq_S_noH_D_RL_Dyno : bpm_dq_S_noH_D_RL_Dyno/bpm_dq_S_noH_D_RL_Dyno  Description=Subsystem: bpm_dq_S_noH_D_RL_Dyno  ic=[0., 0., 0., 0.]  Par1=DualMotor(Load_W).Mechanical.B  Par2=DualMotor(Load_W).Mechanical.Jrotor  Par3=DualMotor(Load_W).Inductance_Variation.Ld_a0  Par4=DualMotor(Load_W).Inductance_Variation.Lq_b0  Par5=2  Par6=DualMotor(Load_W).Electrical.p_Pole_Pairs  Par7=DualMotor(Load_W).Power_Loss.Rot_Loss_Flag  Par8=2  Par9=5  Par10=DualMotor(Load_W).Electrical.Rs_a_Ref  Par11=DualMotor(Load_W).Mechanical.PM_Temperature_Ref  Par12=DualMotor(Load_W).Mechanical.Rs_Temperature_Ref  Par13=DualMotor(Load_W).Electrical.alpha_s  Par14=0.00206  Par15=DualMotor(Load_W).Electrical.PM_Flux_f01  Par16=TimeSteps.ModelStep  Par17=-1.  Par18=-1.  MinStep=1/40
  ia : Outport
  ib : Outport  Port=2
  ic : Outport  Port=3
  OmegaFlux : Outport  Port=4
  OmegaRotMech : Outport  Port=5
  Pmotor : Outport  Port=6
  Tshaft : Outport  Port=7
  Te : Outport  Port=8
  ThetaFlux : Outport  Port=9
  wires:
  bpm_dq_S_noH_D_RL_Dyno/2 -> Terminator8/1
  bpm_dq_S_noH_D_RL_Dyno/1 -> Terminator9/1
  iTDyno/1 -> bpm_dq_S_noH_D_RL_Dyno/6
  Va/1 -> bpm_dq_S_noH_D_RL_Dyno/7
  [oiq] -> Inductance_LUT/2(Iq)
  [oid] -> Inductance_LUT/1(Id)
  bpm_dq_S_noH_D_RL_Dyno/5 -> Terminator5/1
  bpm_dq_S_noH_D_RL_Dyno/7 -> ib/1
  bpm_dq_S_noH_D_RL_Dyno/3 -> Terminator7/1
  bpm_dq_S_noH_D_RL_Dyno/10 -> [oiq]
  bpm_dq_S_noH_D_RL_Dyno/9 -> [oid]
  bpm_dq_S_noH_D_RL_Dyno/8 -> ic/1
  bpm_dq_S_noH_D_RL_Dyno/4 -> Terminator6/1
  Vb/1 -> bpm_dq_S_noH_D_RL_Dyno/8
  Ts/1 -> bpm_dq_S_noH_D_RL_Dyno/4
  Tr/1 -> bpm_dq_S_noH_D_RL_Dyno/3
  bpm_dq_S_noH_D_RL_Dyno/6 -> ia/1
  Vc/1 -> bpm_dq_S_noH_D_RL_Dyno/9
  bpm_dq_S_noH_D_RL_Dyno/11 -> OmegaFlux/1
  bpm_dq_S_noH_D_RL_Dyno/12 -> OmegaRotMech/1, Rot_Loss_LUT/1(omega_m)
  bpm_dq_S_noH_D_RL_Dyno/15 -> Demux/1
  bpm_dq_S_noH_D_RL_Dyno/14 -> Terminator2/1
  bpm_dq_S_noH_D_RL_Dyno/13 -> Terminator3/1
  bpm_dq_S_noH_D_RL_Dyno/16 -> Terminator1/1
  bpm_dq_S_noH_D_RL_Dyno/17 -> Tshaft/1
  bpm_dq_S_noH_D_RL_Dyno/18 -> Te/1
  bpm_dq_S_noH_D_RL_Dyno/20 -> Terminator/1
  bpm_dq_S_noH_D_RL_Dyno/19 -> ThetaFlux/1
  Inductance_LUT/2(LUT_Lq1) -> bpm_dq_S_noH_D_RL_Dyno/2
  Inductance_LUT/1(LUT_Ld1) -> bpm_dq_S_noH_D_RL_Dyno/1
  Rot_Loss_LUT/1(p_rot_loss) -> bpm_dq_S_noH_D_RL_Dyno/5
  Demux/1 -> Terminator4/1
  Demux/2 -> Pmotor/1

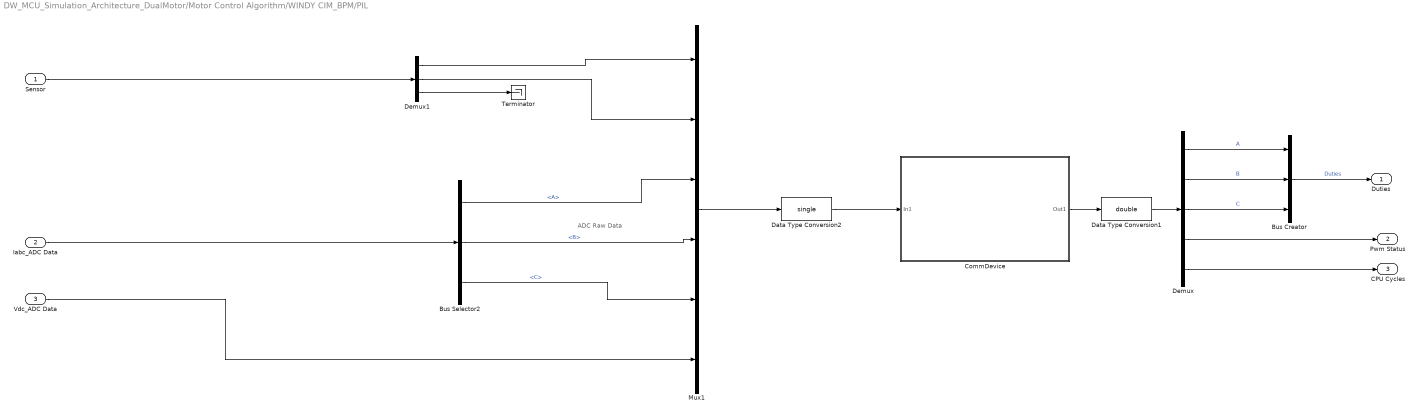
== system DW_MCU_Simulation_Architecture_DualMotor/Motor Control Algorithm/WINDY CIM_BPM/PIL ==
  note: ADC Raw Data
  Sensor : Inport
  Iabc_ADC Data : Inport  Port=2
  Vdc_ADC Data : Inport  Port=3
  Bus Creator : BusCreator  Inputs=3
  Bus Selector2 : BusSelector  OutputSignals=A,B,C
  CommDevice : Subsystem  Variant=on  VariantControl=Variant1
  Data Type Conversion1 : DataTypeConversion  OutDataTypeStr=double
  Data Type Conversion2 : DataTypeConversion  OutDataTypeStr=single
  Demux : Demux  Outputs=5
  Demux1 : Demux  Outputs=3
  Mux1 : Mux  Inputs=6
  Terminator : Terminator
  Duties : Outport
  Pwm Status : Outport  Port=2
  CPU Cycles : Outport  Port=3
  wires:
  Bus Creator/1 -> Duties/1  "Duties"
  Bus Selector2/2 -> Mux1/4  "<B>"
  Bus Selector2/1 -> Mux1/3  "<A>"
  Bus Selector2/3 -> Mux1/5  "<C>"
  Vdc_ADC Data/1 -> Mux1/6
  Iabc_ADC Data/1 -> Bus Selector2/1
  Sensor/1 -> Demux1/1
  Demux1/3 -> Terminator/1
  Demux1/1 -> Mux1/1
  Demux1/2 -> Mux1/2
  Mux1/1 -> Data Type Conversion2/1
  Data Type Conversion2/1 -> CommDevice/1("In1 ")
  Data Type Conversion1/1 -> Demux/1
  Demux/4 -> Pwm Status/1
  Demux/1 -> Bus Creator/1  "A"
  Demux/2 -> Bus Creator/2  "B"
  Demux/3 -> Bus Creator/3  "C"
  CommDevice/1(" Out1") -> Data Type Conversion1/1
  Demux/5 -> CPU Cycles/1

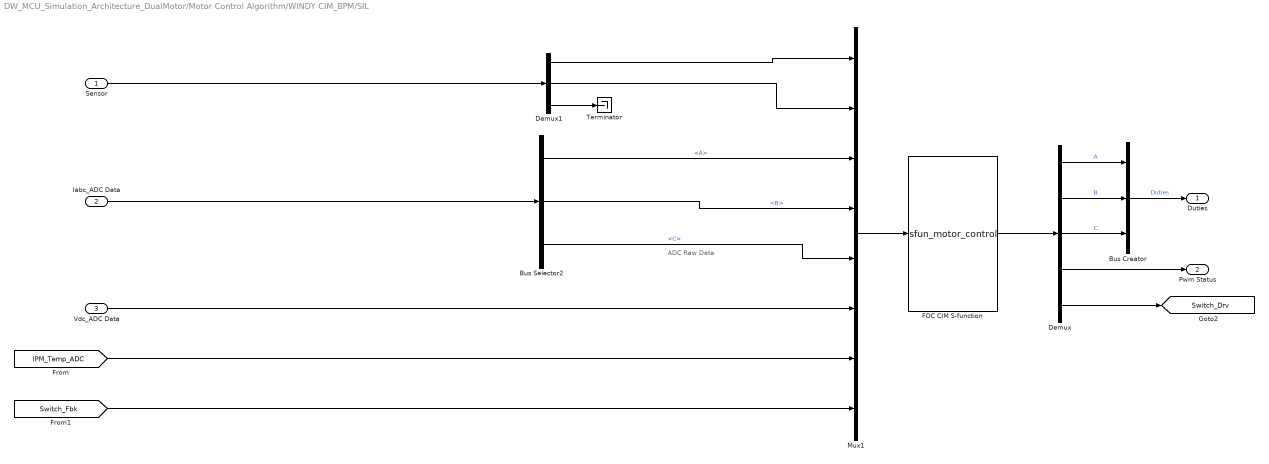
== system DW_MCU_Simulation_Architecture_DualMotor/Motor Control Algorithm/WINDY CIM_BPM/SIL ==
  note: ADC Raw Data
  Sensor : Inport
  Iabc_ADC Data : Inport  Port=2
  Vdc_ADC Data : Inport  Port=3
  Bus Creator : BusCreator  Inputs=3
  Bus Selector2 : BusSelector  OutputSignals=A,B,C
  Demux : Demux  Outputs=5
  Demux1 : Demux  Outputs=3
  "FOC CIM S-function " : S-Function  InitFcn=|  StopFcn=clear CompileStruct;  FunctionName=sfun_motor_control  Parameters=TimeSteps.ModelStep,Paths.Setting_File_Path  SFunctionDeploymentMode=off  EnableBusSupport=off
      | clear mex;
      | CompileStruct.Root_Path_flag=config.Root_Path_flag;
      | CompileStruct.Root_Path=Paths.Root_Path;
      | CompileStruct.Object_Path=Paths.Object_Path;
      | CompileStruct.Fast_ADC_Initialization_Flag=config.Fast_ADC_Initialization_Flag;
      | CompileStruct.Skip_Motor_Moving_Handler_Flag=config.Skip_Motor_Moving_Handler_Flag;
      | CompileStruct.Setting_File_Flag=config.Setting_File_Flag;
      | 
      | if ( (strcmp(get_param('MCU_Simulation_Architecture/config_sub_sys', 'mcu_recompile'), 'on') == 1) || (exist('SimArchUID')==0) || ( strcmp(SimArchUID, 'a') == 0 ) )
      |     Compile_Link_MCU(CompileStruct);
      |     assignin('base', 'SimArchUID', 'a');
      | end
  Mux1 : Mux  Inputs=8
  Terminator : Terminator
  Duties : Outport
  Pwm Status : Outport  Port=2
  tag scope: Switch_Drv=global
  wires:
  Bus Selector2/2 -> Mux1/4  "<B>"
  "FOC CIM S-function "/1 -> Demux/1
  Bus Selector2/1 -> Mux1/3  "<A>"
  Bus Selector2/3 -> Mux1/5  "<C>"
  Vdc_ADC Data/1 -> Mux1/6
  Bus Creator/1 -> Duties/1  "Duties"
  Iabc_ADC Data/1 -> Bus Selector2/1
  Mux1/1 -> "FOC CIM S-function "/1
  Demux1/1 -> Mux1/1
  Demux1/2 -> Mux1/2
  Demux1/3 -> Terminator/1
  Sensor/1 -> Demux1/1
  Demux/1 -> Bus Creator/1  "A"
  Demux/2 -> Bus Creator/2  "B"
  Demux/3 -> Bus Creator/3  "C"
  Demux/4 -> Pwm Status/1
  [IPM_Temp_ADC] -> Mux1/7
  [Switch_Fbk] -> Mux1/8
  Demux/5 -> [Switch_Drv]

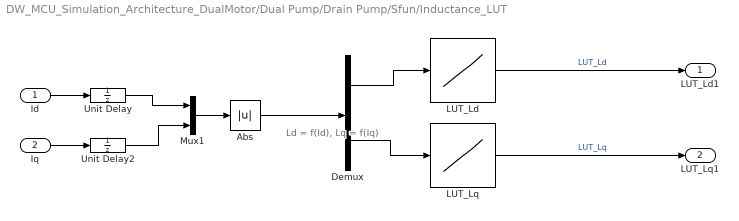
== system DW_MCU_Simulation_Architecture_DualMotor/Dual Pump/Drain Pump/Sfun/Inductance_LUT ==
  note: Ld = f(Id),
      | Lq = f(Iq)
  Id : Inport
  Iq : Inport  Port=2
  Abs : Abs
  Demux : Demux  Outputs=2
  LUT_Ld : Lookup_n-D  NumberOfTableDimensions=1  BreakpointsForDimension1=[DualMotor(Load_D).Inductance_Variation.I_pk0,DualMotor(Load_D).Inductance_Variation.I_pk1,DualMotor(Load_D).Inductance_Variation.I_pk2,DualMotor(Load_D).Inductance_Variation.I_pk3,DualMotor(Load_D).Inductance_Variation.I_pk4,DualMotor(Load_D).Inductance_Variation.I_pk5,DualMotor(Load_D).Inductance_Variation.I_pk6,DualMotor(Load_D).Inductance_Variation.I_pk7]  IndexSearchMethod=Evenly spaced points  Table=[DualMotor(Load_D).Inductance_Variation.Ld_a0,DualMotor(Load_D).Inductance_Variation.Ld_a1,DualMotor(Load_D).Inductance_Variation.Ld_a2,DualMotor(Load_D).Inductance_Variation.Ld_a3,DualMotor(Load_D).Inductance_Variation.Ld_a4,DualMotor(Load_D).Inductance_Variation.Ld_a5,DualMotor(Load_D).Inductance_Variation.Ld_a6,DualMotor(Load_D).Inductance_Variation.Ld_a7]  InternalRulePriority=Speed  RndMeth=Simplest  InputSameDT=on
  LUT_Lq : Lookup_n-D  NumberOfTableDimensions=1  BreakpointsForDimension1=[DualMotor(Load_D).Inductance_Variation.I_pk0,DualMotor(Load_D).Inductance_Variation.I_pk1,DualMotor(Load_D).Inductance_Variation.I_pk2,DualMotor(Load_D).Inductance_Variation.I_pk3,DualMotor(Load_D).Inductance_Variation.I_pk4,DualMotor(Load_D).Inductance_Variation.I_pk5,DualMotor(Load_D).Inductance_Variation.I_pk6,DualMotor(Load_D).Inductance_Variation.I_pk7]  IndexSearchMethod=Evenly spaced points  Table=[DualMotor(Load_D).Inductance_Variation.Lq_b0,DualMotor(Load_D).Inductance_Variation.Lq_b1,DualMotor(Load_D).Inductance_Variation.Lq_b2,DualMotor(Load_D).Inductance_Variation.Lq_b3,DualMotor(Load_D).Inductance_Variation.Lq_b4,DualMotor(Load_D).Inductance_Variation.Lq_b5,DualMotor(Load_D).Inductance_Variation.Lq_b6,DualMotor(Load_D).Inductance_Variation.Lq_b7]  InternalRulePriority=Speed  RndMeth=Simplest  InputSameDT=on
  Mux1 : Mux  Inputs=2
  Unit Delay : UnitDelay  SampleTime=-1
  Unit Delay2 : UnitDelay  SampleTime=-1
  LUT_Ld1 : Outport
  LUT_Lq1 : Outport  Port=2
  wires:
  LUT_Ld/1 -> LUT_Ld1/1  "LUT_Ld"
  Unit Delay/1 -> Mux1/1
  Unit Delay2/1 -> Mux1/2
  Demux/1 -> LUT_Ld/1
  Iq/1 -> Unit Delay2/1
  Abs/1 -> Demux/1
  Mux1/1 -> Abs/1
  Demux/2 -> LUT_Lq/1
  LUT_Lq/1 -> LUT_Lq1/1  "LUT_Lq"
  Id/1 -> Unit Delay/1

== system DW_MCU_Simulation_Architecture_DualMotor/Dual Pump/Drain Pump/Sfun/Rot_Loss_LUT ==
  omega_m : Inport
  Abs : Abs
  Gain : Gain  Gain=9.5493
  Rot_Loss_LUT : Lookup_n-D  NumberOfTableDimensions=1  BreakpointsForDimension1=[DualMotor(Load_D).Power_Loss.Rot_Loss_Speed0,(DualMotor(Load_D).Power_Loss.Rot_Loss_Speed1+0.01),(DualMotor(Load_D).Power_Loss.Rot_Loss_Speed2+0.02),(DualMotor(Load_D).Power_Loss.Rot_Loss_Speed3+0.03),(DualMotor(Load_D).Power_Loss.Rot_Loss_Speed4+0.04),(DualMotor(Load_D).Power_Loss.Rot_Loss_Speed5+0.05),(DualMotor(Load_D).Power_Loss.Rot_Loss_Speed6+0.06),(DualMotor(Load_D).Power_Loss.Rot_Loss_Speed7+0.07)]  IndexSearchMethod=Linear search  Table=[DualMotor(Load_D).Power_Loss.Rot_Loss_Power0,DualMotor(Load_D).Power_Loss.Rot_Loss_Power1,DualMotor(Load_D).Power_Loss.Rot_Loss_Power2,DualMotor(Load_D).Power_Loss.Rot_Loss_Power3,DualMotor(Load_D).Power_Loss.Rot_Loss_Power4,DualMotor(Load_D).Power_Loss.Rot_Loss_Power5,DualMotor(Load_D).Power_Loss.Rot_Loss_Power6,DualMotor(Load_D).Power_Loss.Rot_Loss_Power7]  InternalRulePriority=Speed  RndMeth=Simplest  InputSameDT=on
  Unit Delay : UnitDelay  SampleTime=-1
  p_rot_loss : Outport
  wires:
  Unit Delay/1 -> Rot_Loss_LUT/1
  Abs/1 -> Gain/1
  Gain/1 -> Unit Delay/1
  Rot_Loss_LUT/1 -> p_rot_loss/1
  omega_m/1 -> Abs/1

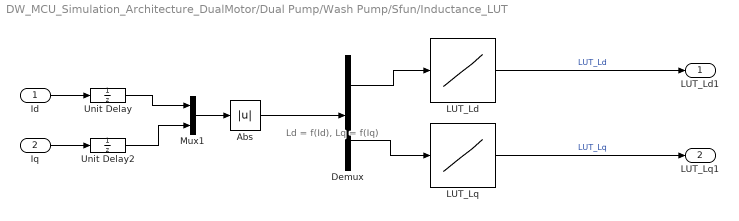
== system DW_MCU_Simulation_Architecture_DualMotor/Dual Pump/Wash Pump/Sfun/Inductance_LUT ==
  note: Ld = f(Id),
      | Lq = f(Iq)
  Id : Inport
  Iq : Inport  Port=2
  Abs : Abs
  Demux : Demux  Outputs=2
  LUT_Ld : Lookup_n-D  NumberOfTableDimensions=1  BreakpointsForDimension1=[DualMotor(Load_W).Inductance_Variation.I_pk0,DualMotor(Load_W).Inductance_Variation.I_pk1,DualMotor(Load_W).Inductance_Variation.I_pk2,DualMotor(Load_W).Inductance_Variation.I_pk3,DualMotor(Load_W).Inductance_Variation.I_pk4,DualMotor(Load_W).Inductance_Variation.I_pk5,DualMotor(Load_W).Inductance_Variation.I_pk6,DualMotor(Load_W).Inductance_Variation.I_pk7]  IndexSearchMethod=Evenly spaced points  Table=[DualMotor(Load_W).Inductance_Variation.Ld_a0,DualMotor(Load_W).Inductance_Variation.Ld_a1,DualMotor(Load_W).Inductance_Variation.Ld_a2,DualMotor(Load_W).Inductance_Variation.Ld_a3,DualMotor(Load_W).Inductance_Variation.Ld_a4,DualMotor(Load_W).Inductance_Variation.Ld_a5,DualMotor(Load_W).Inductance_Variation.Ld_a6,DualMotor(Load_W).Inductance_Variation.Ld_a7]  InternalRulePriority=Speed  RndMeth=Simplest  InputSameDT=on
  LUT_Lq : Lookup_n-D  NumberOfTableDimensions=1  BreakpointsForDimension1=[DualMotor(Load_W).Inductance_Variation.I_pk0,DualMotor(Load_W).Inductance_Variation.I_pk1,DualMotor(Load_W).Inductance_Variation.I_pk2,DualMotor(Load_W).Inductance_Variation.I_pk3,DualMotor(Load_W).Inductance_Variation.I_pk4,DualMotor(Load_W).Inductance_Variation.I_pk5,DualMotor(Load_W).Inductance_Variation.I_pk6,DualMotor(Load_W).Inductance_Variation.I_pk7]  IndexSearchMethod=Evenly spaced points  Table=[DualMotor(Load_W).Inductance_Variation.Lq_b0,DualMotor(Load_W).Inductance_Variation.Lq_b1,DualMotor(Load_W).Inductance_Variation.Lq_b2,DualMotor(Load_W).Inductance_Variation.Lq_b3,DualMotor(Load_W).Inductance_Variation.Lq_b4,DualMotor(Load_W).Inductance_Variation.Lq_b5,DualMotor(Load_W).Inductance_Variation.Lq_b6,DualMotor(Load_W).Inductance_Variation.Lq_b7]  InternalRulePriority=Speed  RndMeth=Simplest  InputSameDT=on
  Mux1 : Mux  Inputs=2
  Unit Delay : UnitDelay  SampleTime=-1
  Unit Delay2 : UnitDelay  SampleTime=-1
  LUT_Ld1 : Outport
  LUT_Lq1 : Outport  Port=2
  wires:
  LUT_Ld/1 -> LUT_Ld1/1  "LUT_Ld"
  Unit Delay/1 -> Mux1/1
  Unit Delay2/1 -> Mux1/2
  Demux/1 -> LUT_Ld/1
  Iq/1 -> Unit Delay2/1
  Abs/1 -> Demux/1
  Mux1/1 -> Abs/1
  Demux/2 -> LUT_Lq/1
  LUT_Lq/1 -> LUT_Lq1/1  "LUT_Lq"
  Id/1 -> Unit Delay/1

== system DW_MCU_Simulation_Architecture_DualMotor/Dual Pump/Wash Pump/Sfun/Rot_Loss_LUT ==
  omega_m : Inport
  Abs : Abs
  Gain : Gain  Gain=9.5493
  Rot_Loss_LUT : Lookup_n-D  NumberOfTableDimensions=1  BreakpointsForDimension1=[DualMotor(Load_W).Power_Loss.Rot_Loss_Speed0,(DualMotor(Load_W).Power_Loss.Rot_Loss_Speed1+0.01),(DualMotor(Load_W).Power_Loss.Rot_Loss_Speed2+0.02),(DualMotor(Load_W).Power_Loss.Rot_Loss_Speed3+0.03),(DualMotor(Load_W).Power_Loss.Rot_Loss_Speed4+0.04),(DualMotor(Load_W).Power_Loss.Rot_Loss_Speed5+0.05),(DualMotor(Load_W).Power_Loss.Rot_Loss_Speed6+0.06),(DualMotor(Load_W).Power_Loss.Rot_Loss_Speed7+0.07)]  IndexSearchMethod=Linear search  Table=[DualMotor(Load_W).Power_Loss.Rot_Loss_Power0,DualMotor(Load_W).Power_Loss.Rot_Loss_Power1,DualMotor(Load_W).Power_Loss.Rot_Loss_Power2,DualMotor(Load_W).Power_Loss.Rot_Loss_Power3,DualMotor(Load_W).Power_Loss.Rot_Loss_Power4,DualMotor(Load_W).Power_Loss.Rot_Loss_Power5,DualMotor(Load_W).Power_Loss.Rot_Loss_Power6,DualMotor(Load_W).Power_Loss.Rot_Loss_Power7]  InternalRulePriority=Speed  RndMeth=Simplest  InputSameDT=on
  Unit Delay : UnitDelay  SampleTime=-1
  p_rot_loss : Outport
  wires:
  Unit Delay/1 -> Rot_Loss_LUT/1
  Abs/1 -> Gain/1
  Gain/1 -> Unit Delay/1
  Rot_Loss_LUT/1 -> p_rot_loss/1
  omega_m/1 -> Abs/1

== system DW_MCU_Simulation_Architecture_DualMotor/Motor Control Algorithm/WINDY CIM_BPM/PIL/CommDevice ==
  "In1 " : Inport
  RS232 : Subsystem  VariantControl=VARIANT_PIL_COMM == 1
  SPI : Subsystem  VariantControl=VARIANT_PIL_COMM == 2
  " Out1" : Outport

== system DW_MCU_Simulation_Architecture_DualMotor/Motor Control Algorithm/WINDY CIM_BPM/PIL/CommDevice/RS232 ==
  In1 : Inport
  PIL_Comm : S-Function  InitFcn=|  FunctionName=serial_sf  Parameters=get_param([bdroot '/serialconfig_ss'], 'com_port'), get_param([bdroot '/serialconfig_ss'], 'baudrate'), steps  SFunctionDeploymentMode=off  EnableBusSupport=off
      | transmission = evalin('base','Motor.Mechanical.TR');
      | spd_blk = [bdroot '/speedcommand_sf']
      | if isempty(get_param(spd_blk,'UserData'))
      | steps = [];
      | else
      |     ud = get_param(spd_blk,'UserData');
      |     [pts,steps] = GenPlotCmds(ud.table);
      |     for i = 1:size(steps,1)
      |         steps(i,1) = steps(i,1) * transmission;
      |         steps(i,2) = steps(i,2) * transmission;
      |     end
      | end
      mask Display:
      | port_label('input', 1, 'Sim Inputs')
      | port_label('output', 1, 'Sim Outputs')
  Out1 : Outport
  wires:
  PIL_Comm/1 -> Out1/1
  In1/1 -> PIL_Comm/1

== system DW_MCU_Simulation_Architecture_DualMotor/Motor Control Algorithm/WINDY CIM_BPM/PIL/CommDevice/SPI ==
  "In1 " : Inport
  S-Function : S-Function  InitFcn=|  FunctionName=cheetah_sf  Parameters=steps  SFunctionDeploymentMode=off  EnableBusSupport=off
      | transmission = evalin('base','Motor.Mechanical.TR');
      | spd_blk = [bdroot '/speedcommand_sf']
      | if isempty(get_param(spd_blk,'UserData'))
      | steps = [];
      | else
      |     ud = get_param(spd_blk,'UserData');
      |     [pts,steps] = GenPlotCmds(ud.table);
      |     for i = 1:size(steps,1)
      |         steps(i,1) = steps(i,1) * transmission;
      |         steps(i,2) = steps(i,2) * transmission;
      |     end
      | end
  " Out1" : Outport
  wires:
  "In1 "/1 -> S-Function/1
  S-Function/1 -> " Out1"/1

== matlab function DW_MCU_Simulation_Architecture_DualMotor/Signal Processing/Direct  Clark  1 ==
  data: XAlphaBeta output Bus: XAlphaBetaBus; Xabc input Bus: XabcBus
function XAlphaBeta = DirectClark(Xabc)

XAlphaBeta.Alpha = Xabc.A;
XAlphaBeta.Beta =  sqrt(3)/3*(Xabc.A+2*Xabc.B);
